simulink model "quarterCar_OpenLoop"  (R2026a)
settings: Solver=VariableStepAuto
undefined symbols (not defined in the file): A, B, C, D

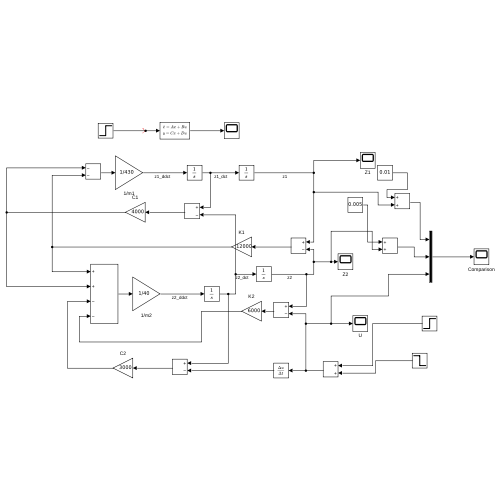
[thumbnail: Simulink's stored preview of the top-level diagram]
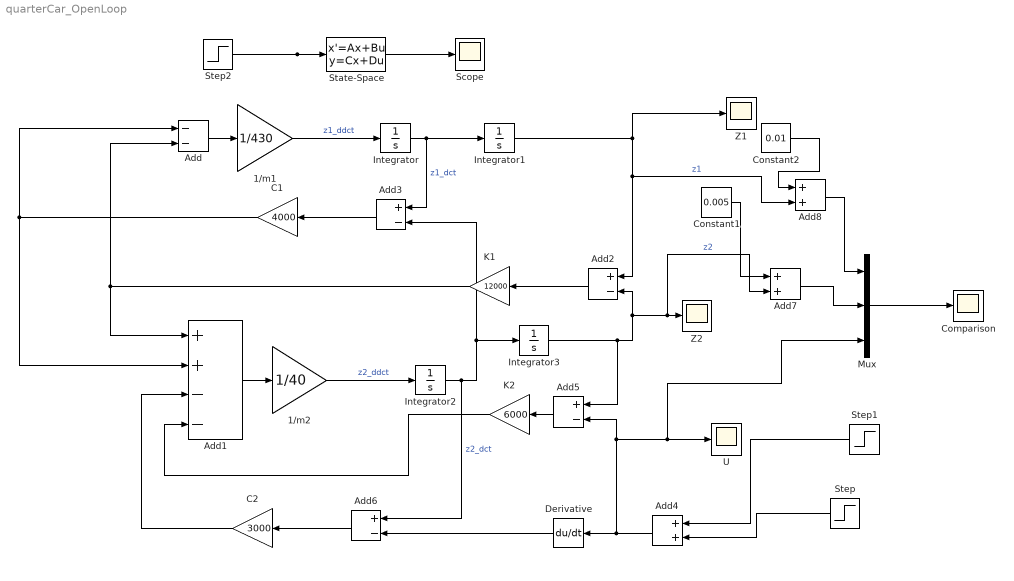
== system quarterCar_OpenLoop ==
  1/m1 : Gain  Gain=1/430
  1/m2 : Gain  Gain=1/40
  Add : Sum  Inputs=--
  Add1 : Sum  Inputs=++--
  Add{2..3,5..6} (4 alike) : Sum  Inputs=+-
  Add4 : Sum
  Add7 : Sum
  Add8 : Sum
  C1 : Gain  Gain=4000
  C2 : Gain  Gain=3000
  Comparison : Scope
      settings: ActiveDisplayYMinimum=-0.002454586518246159  ActiveDisplayYMaximum=0.022091278664215435  DataLoggingVariableName=ScopeData3
  Constant1 : Constant  Value=0.005
  Constant2 : Constant  Value=0.01
  Derivative : Derivative
  Integrator{,1..3} (4 alike) : Integrator
  K1 : Gain  Gain=12000
  K2 : Gain  Gain=6000
  Mux : Mux  Inputs=3
  Scope : Scope
      settings: ActiveDisplayYMinimum=-2.1925451824428435E+77  ActiveDisplayYMaximum=4.7816248449956195E+77  DataLoggingVariableName=ScopeData4
  State-Space : StateSpace  A=A  B=B  C=C  D=D  InitialCondition=0
  Step : Step  Time=4  FinalValue=-0.01  SampleTime=0
  Step1 : Step  Time=3  FinalValue=0.01  SampleTime=0
  Step2 : Step  SampleTime=0
  U : Scope
      settings: ActiveDisplayYMinimum=-0.0012499999999999998  ActiveDisplayYMaximum=0.01125  DataLoggingVariableName=ScopeData2
  Z1 : Scope
      settings: ActiveDisplayYMinimum=-0.0016881753415758619  ActiveDisplayYMaximum=0.010895010755696516
  Z2 : Scope
      settings: ActiveDisplayYMinimum=-0.0013193348765416124  ActiveDisplayYMaximum=0.010361446683257071
  wires:
  1/m1/1 -> Integrator/1  "z1_ddct"
  Integrator/1 -> Add3/1, Integrator1/1  "z1_dct"
  Integrator1/1 -> Add2/1, Add8/2, Z1/1  "z1"
  Add/1 -> 1/m1/1
  1/m2/1 -> Integrator2/1  "z2_ddct"
  Integrator2/1 -> Add6/1, Add3/2, Integrator3/1  "z2_dct"
  Add1/1 -> 1/m2/1
  Integrator3/1 -> Add2/2, Add7/2, Z2/1, Add5/1  "z2"
  Add2/1 -> K1/1
  K1/1 -> Add/2, Add1/1
  Add3/1 -> C1/1
  C1/1 -> Add1/2, Add/1
  Step1/1 -> Add4/1
  Step/1 -> Add4/2
  Add4/1 -> Add5/2, Mux/3, U/1, Derivative/1
  Add5/1 -> K2/1
  K2/1 -> Add1/4
  Add6/1 -> C2/1
  Derivative/1 -> Add6/2
  C2/1 -> Add1/3
  Mux/1 -> Comparison/1
  Constant1/1 -> Add7/1
  Add7/1 -> Mux/2
  Constant2/1 -> Add8/1
  Add8/1 -> Mux/1
  Step2/1 -> State-Space/1
  State-Space/1 -> Scope/1
